simulink library "SyncGenLib"  (R2013a)
settings: Solver=ode45  StartTime=0.0  StopTime=10.0  RelTol=1e-3
libraries: powerlib x16
settings Model: Creator=USER  LastModifiedBy=USER

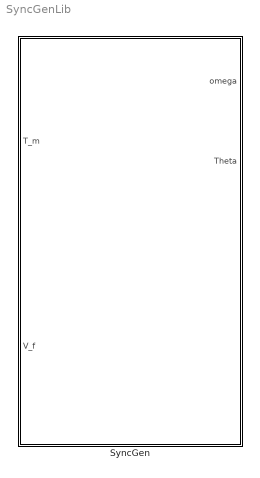
== system SyncGenLib ==
  "SyncGen " : Subsystem  mask{R_f=0.1, R_s=2, D_p=1, J=0.1, M_f=0.5e-2, L_f=1e-2, L_s=1e-2, Omega_0=0, Theta_0=0}
      mask prompts: R_f "Value of the rotor resistor"; R_s "Value of the stator resistor"; D_p "The viscose frection droop factor"; J "Rotor momont of inertia"; M_f "The rotror-stator inductance factor"; L_f "The rotor inductance factor"; L_s "The stator inductance factor"
      mask help: Sync generator with no assumptions.

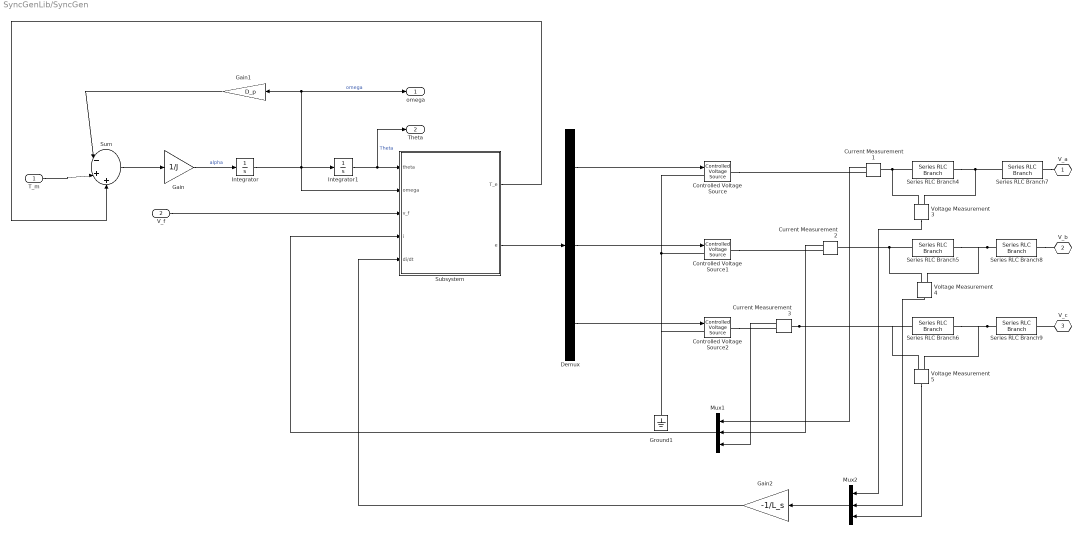
== system SyncGenLib/SyncGen  ==
  T_m : Inport
  V_f : Inport  Port=2
  Controlled Voltage Source : powerlib/Electrical Sources/Controlled Voltage Source  Initialize=off  Source_Type=AC  Amplitude=0  Phase=0  Frequency=0  Measurements=None
  Controlled Voltage Source1 : powerlib/Electrical Sources/Controlled Voltage Source  Initialize=off  Source_Type=AC  Amplitude=0  Phase=0  Frequency=0  Measurements=None
  Controlled Voltage Source2 : powerlib/Electrical Sources/Controlled Voltage Source  Initialize=off  Source_Type=AC  Amplitude=0  Phase=0  Frequency=0  Measurements=None
  Current Measurement1 : powerlib/Measurements/Current Measurement  PhasorSimulation=off  OutputType=Complex  PSBequivalent=0
  Current Measurement2 : powerlib/Measurements/Current Measurement  PhasorSimulation=off  OutputType=Complex  PSBequivalent=0
  Current Measurement3 : powerlib/Measurements/Current Measurement  PhasorSimulation=off  OutputType=Complex  PSBequivalent=0
  Demux : Demux  Outputs=3
  Gain : Gain  Gain=1/J
  Gain1 : Gain  Gain=D_p
  Gain2 : Gain  Gain=-1/L_s
  Ground1 : powerlib/Elements/Ground  LConnTagsString=a
  Integrator : Integrator  InitialCondition=Omega_0
  Integrator1 : Integrator  InitialCondition=Theta_0
  Mux1 : Mux  Inputs=3
  Mux2 : Mux  Inputs=3
  Series RLC Branch4 : powerlib/Elements/Series RLC Branch  LConnTagsString=__new0  RConnTagsString=__new0  BranchType=L  Resistance=R_s  Inductance=L_s  SetiL0=off  InitialCurrent=0  Capacitance=1e-6  Setx0=off  InitialVoltage=0  Measurements=None
  Series RLC Branch5 : powerlib/Elements/Series RLC Branch  LConnTagsString=__new0  RConnTagsString=__new0  BranchType=L  Resistance=R_s  Inductance=L_s  SetiL0=off  InitialCurrent=0  Capacitance=1e-6  Setx0=off  InitialVoltage=0  Measurements=None
  Series RLC Branch6 : powerlib/Elements/Series RLC Branch  LConnTagsString=__new0  RConnTagsString=__new0  BranchType=L  Resistance=R_s  Inductance=L_s  SetiL0=off  InitialCurrent=0  Capacitance=1e-6  Setx0=off  InitialVoltage=0  Measurements=None
  Series RLC Branch7 : powerlib/Elements/Series RLC Branch  LConnTagsString=__new0  RConnTagsString=__new0  BranchType=R  Resistance=R_s  Inductance=L_s  SetiL0=off  InitialCurrent=0  Capacitance=1e-6  Setx0=off  InitialVoltage=0  Measurements=None
  Series RLC Branch8 : powerlib/Elements/Series RLC Branch  LConnTagsString=__new0  RConnTagsString=__new0  BranchType=R  Resistance=R_s  Inductance=L_s  SetiL0=off  InitialCurrent=0  Capacitance=1e-6  Setx0=off  InitialVoltage=0  Measurements=None
  Series RLC Branch9 : powerlib/Elements/Series RLC Branch  LConnTagsString=__new0  RConnTagsString=__new0  BranchType=R  Resistance=R_s  Inductance=L_s  SetiL0=off  InitialCurrent=0  Capacitance=1e-6  Setx0=off  InitialVoltage=0  Measurements=None
  Subsystem : Subsystem
  Sum : Sum  Inputs=|-++
  Voltage Measurement3 : powerlib/Measurements/Voltage Measurement  PhasorSimulation=off  OutputType=Complex  PSBequivalent=0
  Voltage Measurement4 : powerlib/Measurements/Voltage Measurement  PhasorSimulation=off  OutputType=Complex  PSBequivalent=0
  Voltage Measurement5 : powerlib/Measurements/Voltage Measurement  PhasorSimulation=off  OutputType=Complex  PSBequivalent=0
  V_a : PMIOPort  Tag=PMCPort  Port=1  Side=Right
  V_b : PMIOPort  Tag=PMCPort  Port=2  Side=Right
  V_c : PMIOPort  Tag=PMCPort  Port=3  Side=Right
  omega : Outport
  Theta : Outport  Port=2
  wires:
  Sum/1 -> Gain/1
  Gain/1 -> Integrator/1  "alpha"
  Integrator/1 -> Subsystem/2(omega), omega/1, Gain1/1, Integrator1/1  "omega"
  Gain1/1 -> Sum/1
  T_m/1 -> Sum/2
  Integrator1/1 -> Theta/1, Subsystem/1("theta ")  "Theta"
  Demux/1 -> Controlled Voltage Source/1
  Demux/2 -> Controlled Voltage Source1/1
  Demux/3 -> Controlled Voltage Source2/1
  Subsystem/1("T_e ") -> Sum/3
  Current Measurement1/1 -> Mux1/1
  Current Measurement2/1 -> Mux1/2
  Current Measurement3/1 -> Mux1/3
  Mux1/1 -> Subsystem/4(i)
  Subsystem/2(e) -> Demux/1
  Voltage Measurement3/1 -> Mux2/1
  Voltage Measurement4/1 -> Mux2/2
  Voltage Measurement5/1 -> Mux2/3
  Mux2/1 -> Gain2/1
  Gain2/1 -> Subsystem/5(di/dt)
  V_f/1 -> Subsystem/3(v_f)
  connections:
  Controlled Voltage Source/LConn1 -- Controlled Voltage Source1/LConn1 -- Controlled Voltage Source2/LConn1 -- Ground1/LConn1
  Series RLC Branch4/LConn1 -- Voltage Measurement3/LConn1 -- Current Measurement1/LConn1
  Voltage Measurement4/LConn1 -- Series RLC Branch5/LConn1 -- Current Measurement2/LConn1
  Current Measurement3/LConn1 -- Series RLC Branch6/LConn1 -- Voltage Measurement5/LConn1
  Voltage Measurement3/LConn2 -- Series RLC Branch4/RConn1 -- Series RLC Branch7/LConn1
  Series RLC Branch8/LConn1 -- Series RLC Branch5/RConn1 -- Voltage Measurement4/LConn2
  Series RLC Branch9/LConn1 -- Series RLC Branch6/RConn1 -- Voltage Measurement5/LConn2
  Controlled Voltage Source/RConn1 -- Current Measurement1/RConn1
  Controlled Voltage Source1/RConn1 -- Current Measurement2/RConn1
  Controlled Voltage Source2/RConn1 -- Current Measurement3/RConn1
  Series RLC Branch7/RConn1 -- V_a/RConn1
  Series RLC Branch8/RConn1 -- V_b/RConn1
  V_c/RConn1 -- Series RLC Branch9/RConn1

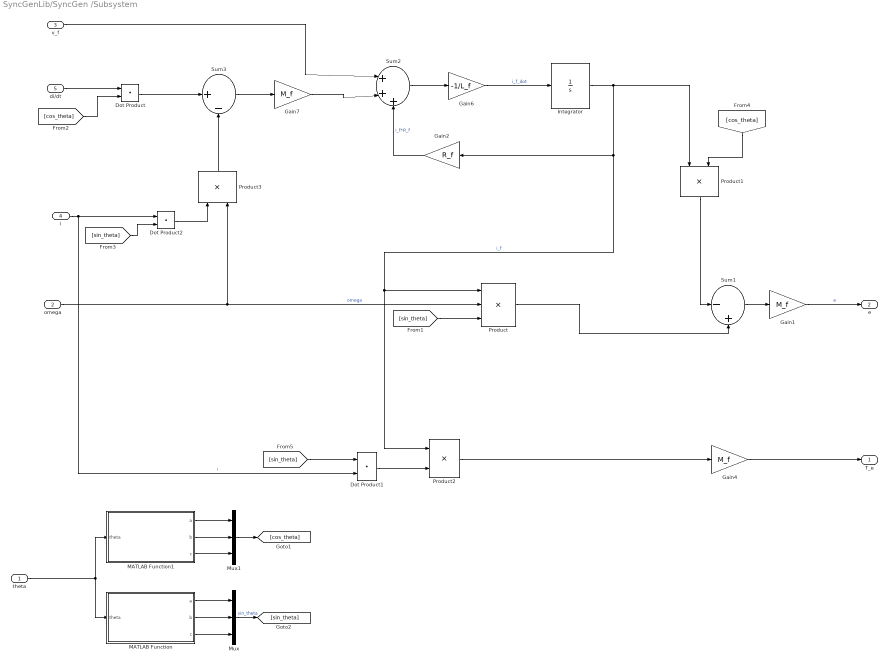
== system SyncGenLib/SyncGen /Subsystem ==
  "theta " : Inport  OutDataTypeStr=double
  omega : Inport  Port=2
  v_f : Inport  Port=3
  i : Inport  Port=4
  di/dt : Inport  Port=5
  Dot Product : DotProduct  InputSameDT=on  OutDataTypeStr=Inherit: Inherit via internal rule
  Dot Product1 : DotProduct  InputSameDT=on  OutDataTypeStr=Inherit: Inherit via internal rule
  Dot Product2 : DotProduct  InputSameDT=on  OutDataTypeStr=Inherit: Inherit via internal rule
  Gain1 : Gain  Gain=M_f
  Gain2 : Gain  Gain=R_f
  Gain4 : Gain  Gain=M_f
  Gain6 : Gain  Gain=-1/L_f
  Gain7 : Gain  Gain=M_f
  Integrator : Integrator
  MATLAB Function : MATLAB Function  TreatAsAtomicUnit=on
  MATLAB Function1 : MATLAB Function  TreatAsAtomicUnit=on
  Mux : Mux  Inputs=3
  Mux1 : Mux  Inputs=3
  Product : Product  Inputs=3
  Product1 : Product
  Product2 : Product
  Product3 : Product
  Sum1 : Sum  Inputs=|-+
  Sum2 : Sum  Inputs=|+++
  Sum3 : Sum  Inputs=|+-
  "T_e " : Outport
  e : Outport  Port=2
  wires:
  Gain1/1 -> e/1  "e"
  MATLAB Function/1(a) -> Mux/1
  MATLAB Function/2(b) -> Mux/2
  MATLAB Function/3(c) -> Mux/3
  Integrator/1 -> Product2/1, Product/1, Gain2/1, Product1/1  "i_f"
  MATLAB Function1/1(a) -> Mux1/1
  MATLAB Function1/2(b) -> Mux1/2
  MATLAB Function1/3(c) -> Mux1/3
  Dot Product/1 -> Sum3/1
  i/1 -> Dot Product2/1, Dot Product1/2  "i"
  "theta "/1 -> MATLAB Function/1(theta), MATLAB Function1/1(theta)
  omega/1 -> Product3/2, Product/2  "omega"
  Dot Product1/1 -> Product2/2
  Product2/1 -> Gain4/1
  Sum3/1 -> Gain7/1
  Dot Product2/1 -> Product3/1
  Product3/1 -> Sum3/2
  di/dt/1 -> Dot Product/1
  v_f/1 -> Sum2/1
  Mux1/1 -> [cos_theta]
  Mux/1 -> [sin_theta]  "sin_theta"
  [sin_theta] -> Product/3
  [cos_theta] -> Dot Product/2
  [sin_theta] -> Dot Product2/2
  Gain7/1 -> Sum2/2
  Gain2/1 -> Sum2/3  "i_f*R_f"
  Sum2/1 -> Gain6/1
  Gain6/1 -> Integrator/1  "i_f_dot"
  Product/1 -> Sum1/2
  Product1/1 -> Sum1/1
  [cos_theta] -> Product1/2
  Sum1/1 -> Gain1/1
  [sin_theta] -> Dot Product1/1
  Gain4/1 -> "T_e "/1

== matlab function SyncGenLib/SyncGen /Subsystem/MATLAB Function ==
  data: theta input; a output; b output; c output
function [a, b, c] = sin_theta(theta)
a = sin(theta);
b = sin(theta -2*pi/3);
c = sin(theta -4*pi/3);

== matlab function SyncGenLib/SyncGen /Subsystem/MATLAB Function1 ==
  data: theta input; a output; b output; c output
function [a, b, c] = cos_theta(theta)
a = cos(theta);
b = cos(theta -2*pi/3);
c = cos(theta -4*pi/3);
